simulink model "T3bloques"  (R2025a)
settings: Solver=VariableStepAuto  StartTime=0.0  StopTime=10.0  RelTol=1e-3
InitFcn:
  | m1 = 290;
  | b1 = 1000;
  | m2 = 59;
  | k1 = 16182;
  | f = 0;
  | k2 = 19000;
settings Model: Creator=carlo  LastModifiedBy=carlo

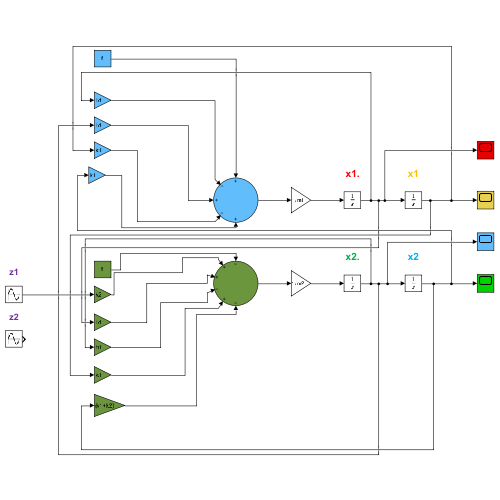
[thumbnail: Simulink's stored preview of the top-level diagram]
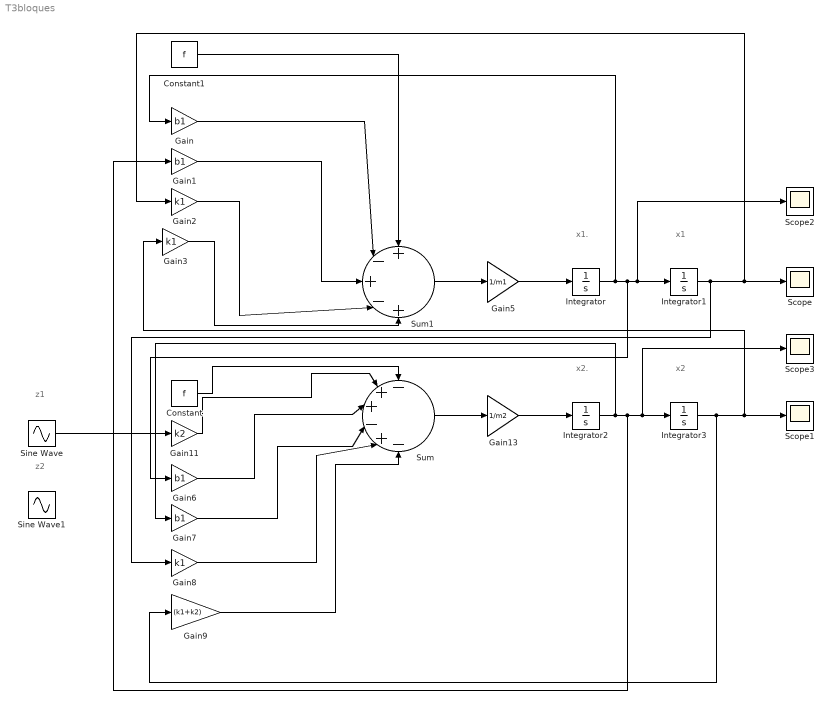
== system T3bloques ==
  note: x1.
  note: x1
  note: x2.
  note: x2
  note: z1
  note: z2
  Constant : Constant  Value=f
  Constant1 : Constant  Value=f
  Gain{,1,6..7} (4 alike) : Gain  Gain=b1
  Gain11 : Gain  Gain=k2
  Gain13 : Gain  Gain=1/m2
  Gain2 : Gain  Gain=k1
  Gain3 : Gain  Gain=k1
  Gain5 : Gain  Gain=1/m1
  Gain8 : Gain  Gain=k1
  Gain9 : Gain  Gain=(k1+k2)
  Integrator{,1..3} (4 alike) : Integrator
  Scope{,1..3} (4 alike) : Scope
      Scope settings: ActiveDisplayYMinimum=-1  ActiveDisplayYMaximum=1
      Scope1 settings: ActiveDisplayYMinimum=-0.066392429182942844  ActiveDisplayYMaximum=0.070956552851740851
      Scope2 settings: ActiveDisplayYMinimum=-0.14350753834021374  ActiveDisplayYMaximum=0.16138258231429412  DataLoggingVariableName=ScopeData2
      Scope3 settings: ActiveDisplayYMinimum=-0.070240527704496708  ActiveDisplayYMaximum=0.080554855938756692  DataLoggingVariableName=ScopeData3
  Sine Wave : Sin  Amplitude=0.05  Frequency=0.5*pi  SampleTime=0
  Sine Wave1 : Sin  Amplitude=0.05  Frequency=20*pi  SampleTime=0
  Sum : Sum  Inputs=-++-+-
  Sum1 : Sum  Inputs=+-+-+
  wires:
  Sum1/1 -> Gain5/1
  Gain5/1 -> Integrator/1
  Integrator/1 -> Gain/1, Gain6/1, Scope2/1, Integrator1/1
  Integrator1/1 -> Gain8/1, Scope/1, Gain2/1
  Sum/1 -> Gain13/1
  Gain13/1 -> Integrator2/1
  Integrator2/1 -> Gain7/1, Gain1/1, Scope3/1, Integrator3/1
  Integrator3/1 -> Gain9/1, Gain3/1, Scope1/1
  Constant1/1 -> Sum1/1
  Gain/1 -> Sum1/2
  Gain1/1 -> Sum1/3
  Gain2/1 -> Sum1/4
  Gain3/1 -> Sum1/5
  Constant/1 -> Sum/1
  Gain11/1 -> Sum/2
  Gain6/1 -> Sum/3
  Gain7/1 -> Sum/4
  Gain8/1 -> Sum/5
  Gain9/1 -> Sum/6
  Sine Wave/1 -> Gain11/1
